simulink model "mech_stewart_js"  (Simulink 7.1)
settings: Solver=ode45  StartTime=0.0  StopTime=inf  RelTol=1e-3
PreLoadFcn:
  | mech_stewartplatform_dat
PostLoadFcn:
  | find_system(gcs,'FollowLinks', 'on', 'LookUnderMasks', 'all');
InitFcn:
  | find_system(gcs,'FollowLinks', 'on', 'LookUnderMasks', 'all');
values from neighbouring files (symbols this model uses):
  body_pts = pos_top' - height*[zeros(2,6);ones(1,6)]    [mech_stewart_studies_setup.m]    (also in mech_stewartplatform_dat.m)
  height = 2.0    (= 2)    [mech_stewart_studies_setup.m]    (also in mech_stewartplatform_dat.m)
  Kd = 4.5e4    (= 45000)    [mech_stewart_studies_setup.m]    (also in mech_stewartplatform_dat.m)
  Ki = 1e4    (= 10000)    [mech_stewart_studies_setup.m]    (also in mech_stewartplatform_dat.m)
  Kp = 2e6    (= 2000000)    [mech_stewart_studies_setup.m]    (also in mech_stewartplatform_dat.m)
  pos_base = []    [mech_stewart_studies_setup.m]    (also in mech_stewartplatform_dat.m)
  pos_top = [pos_top(6,:); pos_top(1:5,:)]    [mech_stewart_studies_setup.m]    (also in mech_stewartplatform_dat.m)
undefined symbols (not defined in the file or in its folder): lower_leg_mass, top_inertia, top_mass, upper_leg_mass
libraries: mblibv1 x9, simulink x6, mech_stewartplatform_leg x6, vrlib x1
Description:
  | Stewart Platform with Joystick Control
  | 
  | Stewart platform with external virtual reality joystick control.
settings Model: Creator=jwendlan  LastModifiedBy=batserve  ExtModeAutoUpdateStatusClock=off
settings DataIOCC: SignalLoggingName=sigsOut  OutputTimes=[0:0.01:50]
settings OptimizationCC: BooleanDataType=off  InlineInvariantSignals=on
settings DebuggingCC: SaveWithParameterizedLinksMsg=none  CheckExecutionContextPreStartOutputMsg=on  CheckExecutionContextRuntimeOutputMsg=on  SignalResolutionControl=TryResolveAllWithWarning  SolverPrmCheckMsg=none  MultiTaskDSMMsg=warning  MultiTaskCondExecSysMsg=none  SigSpecEnsureSampleTimeMsg=none  UnconnectedOutputMsg=none  StrictBusMsg=None
settings HardwareCC: TargetBitPerLong=64  TargetEndianess=LittleEndian  TargetWordSize=64  TargetHWDeviceType=MATLAB Host  ProdEqTarget=off
settings RTWCC: SystemTargetFile=rsim.tlc  TemplateMakefile=rsim_default_tmf  Description=Rapid Simulation Target  ProcessScript=rsim_make_rtw_hook  IncludeERTFirstTime=on
settings RSimTargetCC: TargetFcnLib=ansi_tfl_tmw.mat  TargetFunctionLibrary=ANSI_C  IsPILTarget=off  EnableShiftOperators=on  PortableWordSizes=off
settings SimMechanicsCC: VisOnUpdateDiagram=on  VisDuringSimulation=on

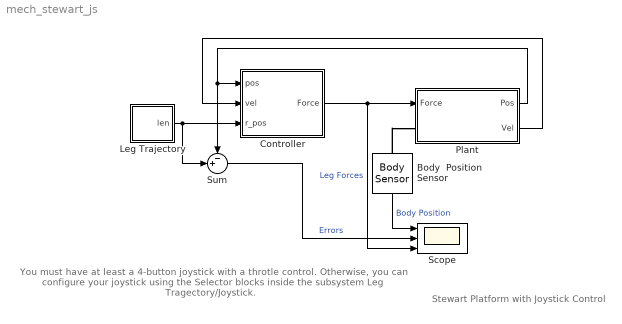
== system mech_stewart_js ==
  note: Stewart Platform
      | with Joystick Control
  note: You must have at least a 4-button
      | joystick with a throtle control.
      | Otherwise, you can configure
      | your joystick using the Selector
      | blocks inside the subsystem
      | Leg Tragectory/Joystick.
  Body  Position Sensor : mblibv1/Sensors &  Actuators/Body Sensor  Orientation=down  DialogController=MECH.DynMechDlgSource  SystemSampleTime=-1  PhysicalDomain=Mechanical  PortType=blob  Muxed=on  Pose=off  Angle=on  AngleUnits=deg  ArcVelocity=off  ArcVelocityUnits=deg/s  ArcAcceleration=off  ArcAccelerationUnits=deg/s^2  CoordPosition=on  CoordPositionUnits=m  Velocity=off  VelocityUnits=m/s  Acceleration=off  AccelerationUnits=m/s^2  Quaternion=on  QuaternionDT=off  QuaternionDDT=off  QuaternionUnits=off  OutputVector=[ 3 ]  ActiveIO=on  Width=3  DialogClass=MechanicalSensorBlock  ReferenceFrame=Absolute (World)
  Controller : Subsystem
  Leg Trajectory : Subsystem
  Plant : Subsystem
  Scope : Scope  NumInputPorts=3
      settings: Tag=OpenMeAtStartUp  YMin=-1~-1.1~-20000  YMax=3.5~1.1~40000
  Sum : Sum  Inputs=-+|  OutDataType=sfix(16)  OutScaling=2^0  SaturateOnIntegerOverflow=on  InputSameDT=on  OutDataTypeStr=Inherit: Same as first input
  wires:
  Controller/1(Force) -> Plant/1(Force), Scope/3  "Leg Forces"
  Body  Position Sensor/1 -> Scope/1  "Body Position"
  Sum/1 -> Scope/2  "Errors"
  Leg Trajectory/1(len) -> Controller/3(r_pos), Sum/2
  Plant/2(Vel) -> Controller/2(vel)
  Plant/1(Pos) -> Controller/1(pos), Sum/1
  connections:
  Body  Position Sensor/LConn1 -- Plant/LConn1

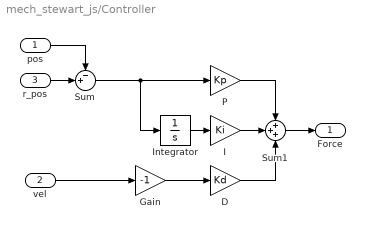
== system mech_stewart_js/Controller ==
  pos : Inport  OutDataType=sfix(16)  OutScaling=2^0
  vel : Inport  Port=2  OutDataType=sfix(16)  OutScaling=2^0
  r_pos : Inport  Port=3  OutDataType=sfix(16)  OutScaling=2^0
  D : Gain  Gain=Kd  ParameterDataType=sfix(16)  ParameterScaling=2^0  OutDataType=sfix(16)  OutScaling=2^0  SaturateOnIntegerOverflow=on  OutDataTypeStr=Inherit: Same as input  ParamDataTypeStr=Inherit: Same as input
  Gain : Gain  Gain=-1  ParameterDataType=sfix(16)  ParameterScaling=2^0  OutDataType=sfix(16)  OutScaling=2^0  SaturateOnIntegerOverflow=on  OutDataTypeStr=Inherit: Same as input  ParamDataTypeStr=Inherit: Same as input
  I : Gain  Gain=Ki  ParameterDataType=sfix(16)  ParameterScaling=2^0  OutDataType=sfix(16)  OutScaling=2^0  SaturateOnIntegerOverflow=on  OutDataTypeStr=Inherit: Same as input  ParamDataTypeStr=Inherit: Same as input
  Integrator : Integrator  InitialCondition=(upper_leg_mass+lower_leg_mass+(top_mass*1.3/6))*9.81/Ki  ZeroCross=off
  P : Gain  Gain=Kp  ParameterDataType=sfix(16)  ParameterScaling=2^0  OutDataType=sfix(16)  OutScaling=2^0  SaturateOnIntegerOverflow=on  OutDataTypeStr=Inherit: Same as input  ParamDataTypeStr=Inherit: Same as input
  Sum : Sum  Inputs=-+|  OutDataType=sfix(16)  OutScaling=2^0  SaturateOnIntegerOverflow=on  InputSameDT=on  OutDataTypeStr=Inherit: Same as first input
  Sum1 : Sum  Inputs=+++  OutDataType=sfix(16)  OutScaling=2^0  SaturateOnIntegerOverflow=on  InputSameDT=on  OutDataTypeStr=Inherit: Same as first input
  Force : Outport  OutDataType=sfix(16)  OutScaling=2^0
  wires:
  Sum/1 -> P/1, Integrator/1
  I/1 -> Sum1/2
  P/1 -> Sum1/1
  Integrator/1 -> I/1
  vel/1 -> Gain/1
  D/1 -> Sum1/3
  pos/1 -> Sum/1
  Sum1/1 -> Force/1
  r_pos/1 -> Sum/2
  Gain/1 -> D/1

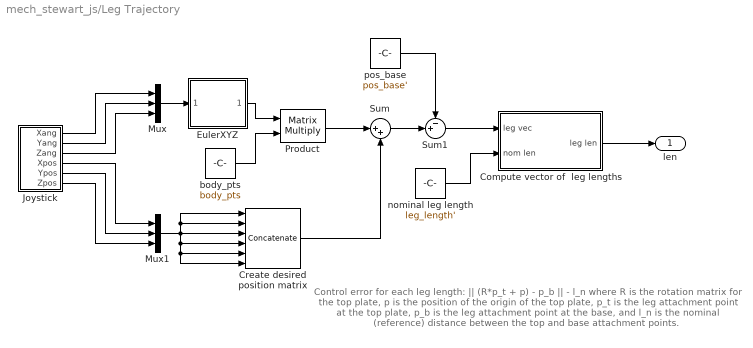
== system mech_stewart_js/Leg Trajectory ==
  note: Control error for each leg length:
      |
      |   || (R*p_t + p) - p_b || - l_n
      |
      | where R is the rotation matrix
      | for the top plate, p is the position
      | of the origin of the top plate, p_t
      | is the leg attachment point at the
      | top plate, p_b is the leg attachment
      | point at the base, and l_n is the
      | nominal (reference) distance between
      | the top and base attachment points.
  Compute vector of  leg lengths : Subsystem  TreatAsAtomicUnit=on
  Create desired position matrix : Concatenate  NumInputs=6  Mode=Multidimensional array  ConcatenateDimension=2
  EulerXYZ : Subsystem
      mask Type: EulerXYZ
      mask Description: Creates the EulerXYZ rotation matrix corresponding to body fixed rotations in the X, Y, and then Z. This matrix maps body vectors to world vectors.
      mask Help:
      | <p>This block determines the EulerXYZ matrix from a 3x1 euler angles in the X, Y, & Z directions. The matrix maps vectors the body axes to the inertial axes.</p>
      | 
      | <p>The block input and output contain more than one signal as described below.</p>
      | 
      | <p><H4>Block Vector Input - Euler XYZ angles</H4>
      |     <ul>
      |     <li>X angle</li>
      |     <li>Y angle</li>
      |     <li>Z angle</li>
      |    </ul>
      |    </p>
      | 
      | <p><H4>Block Matrix Output - XYZ Euler Matrix </H4>
      |     <ul>
      |    </ul>
      |    </p>
      mask Display: disp('Rotation\nMatrix')
  Joystick : Subsystem
  Mux : Mux  Inputs=3
  Mux1 : Mux  Inputs=3
  Product : Product  Multiplication=Matrix(*)  OutDataType=sfix(16)  OutScaling=2^0  SaturateOnIntegerOverflow=on  InputSameDT=on  OutDataTypeStr=Inherit: Same as first input
  Sum : Sum  Inputs=|++  OutDataType=sfix(16)  OutScaling=2^0  SaturateOnIntegerOverflow=on  InputSameDT=on  OutDataTypeStr=Inherit: Same as first input
  Sum1 : Sum  Inputs=-+|  OutDataType=sfix(16)  OutScaling=2^0  SaturateOnIntegerOverflow=on  InputSameDT=on  OutDataTypeStr=Inherit: Same as first input
  body_pts : Constant  Value=body_pts  VectorParams1D=off  OutDataType=sfix(16)  OutScaling=2^0
  nominal leg length : Constant  Value=leg_length'  VectorParams1D=off  OutDataType=sfix(16)  OutScaling=2^0
  pos_base : Constant  Value=pos_base'  VectorParams1D=off  OutDataType=sfix(16)  OutScaling=2^0
  len : Outport  OutDataType=sfix(16)  OutScaling=2^0
  wires:
  Joystick/6(Zpos) -> Mux1/3
  Joystick/5(Ypos) -> Mux1/2
  Joystick/4(Xpos) -> Mux1/1
  Joystick/2(Yang) -> Mux/2
  Joystick/1(Xang) -> Mux/1
  Joystick/3(Zang) -> Mux/3
  Compute vector of  leg lengths/1(leg len) -> len/1
  nominal leg length/1 -> Compute vector of  leg lengths/2(nom len)
  Sum1/1 -> Compute vector of  leg lengths/1(leg vec)
  Sum/1 -> Sum1/2
  pos_base/1 -> Sum1/1
  Create desired position matrix/1 -> Sum/2
  Mux1/1 -> Create desired position matrix/6, Create desired position matrix/5, Create desired position matrix/4, Create desired position matrix/2, Create desired position matrix/1, Create desired position matrix/3
  Product/1 -> Sum/1
  body_pts/1 -> Product/2
  EulerXYZ/1(EulerXYZ) -> Product/1
  Mux/1 -> EulerXYZ/1(x y z angles)

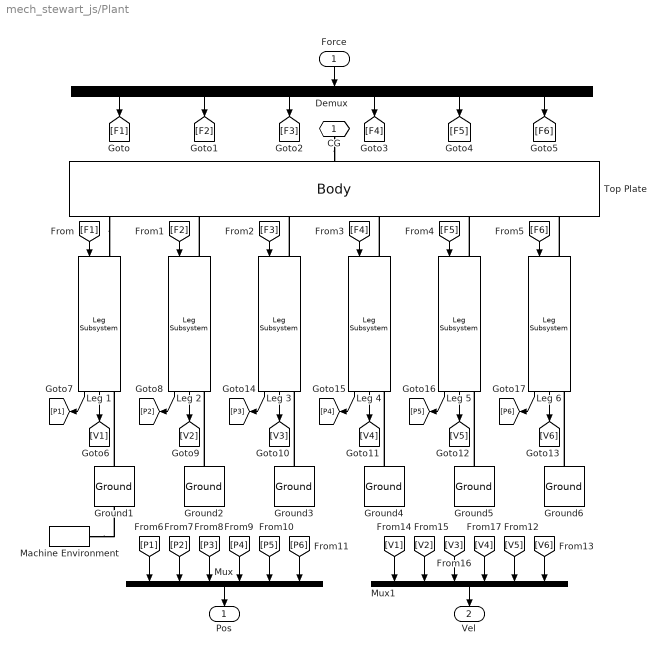
== system mech_stewart_js/Plant ==
  Force : Inport  Orientation=down  OutDataType=sfix(16)  OutScaling=2^0
  Demux : Demux  Orientation=down  Outputs=6
  Ground1 : mblibv1/Bodies/Ground  Orientation=up  DialogController=MECH.DynMechDlgSource  SystemSampleTime=-1  LeftPortType=env  RightPortType=workingframe  PhysicalDomain=Mechanical  DialogClass=GroundBlock  CoordPosition=pos_base(1,:)  CoordPositionUnits=m  StateVectorMgrId=-1  MachineId=[0 0]  ShowEnvPort=on
  Ground2 : mblibv1/Bodies/Ground  Orientation=up  DialogController=MECH.DynMechDlgSource  SystemSampleTime=-1  LeftPortType=env  RightPortType=workingframe  PhysicalDomain=Mechanical  DialogClass=GroundBlock  CoordPosition=pos_base(2,:)  CoordPositionUnits=m  StateVectorMgrId=-1  MachineId=[0 0]  ShowEnvPort=off
  Ground3 : mblibv1/Bodies/Ground  Orientation=up  DialogController=MECH.DynMechDlgSource  SystemSampleTime=-1  LeftPortType=env  RightPortType=workingframe  PhysicalDomain=Mechanical  DialogClass=GroundBlock  CoordPosition=pos_base(3,:)  CoordPositionUnits=m  StateVectorMgrId=-1  MachineId=[0 0]  ShowEnvPort=off
  Ground4 : mblibv1/Bodies/Ground  Orientation=up  DialogController=MECH.DynMechDlgSource  SystemSampleTime=-1  LeftPortType=env  RightPortType=workingframe  PhysicalDomain=Mechanical  DialogClass=GroundBlock  CoordPosition=pos_base(4,:)  CoordPositionUnits=m  StateVectorMgrId=-1  MachineId=[0 0]  ShowEnvPort=off
  Ground5 : mblibv1/Bodies/Ground  Orientation=up  DialogController=MECH.DynMechDlgSource  SystemSampleTime=-1  LeftPortType=env  RightPortType=workingframe  PhysicalDomain=Mechanical  DialogClass=GroundBlock  CoordPosition=pos_base(5,:)  CoordPositionUnits=m  StateVectorMgrId=-1  MachineId=[0 0]  ShowEnvPort=off
  Ground6 : mblibv1/Bodies/Ground  Orientation=up  DialogController=MECH.DynMechDlgSource  SystemSampleTime=-1  LeftPortType=env  RightPortType=workingframe  PhysicalDomain=Mechanical  DialogClass=GroundBlock  CoordPosition=pos_base(6,:)  CoordPositionUnits=m  StateVectorMgrId=-1  MachineId=[0 0]  ShowEnvPort=off
  Leg 1 : mech_stewartplatform_leg/Leg Subsystem  Orientation=down  SystemSampleTime=-1  ln=1
  Leg 2 : mech_stewartplatform_leg/Leg Subsystem  Orientation=down  SystemSampleTime=-1  ln=2
  Leg 3 : mech_stewartplatform_leg/Leg Subsystem  Orientation=down  SystemSampleTime=-1  ln=3
  Leg 4 : mech_stewartplatform_leg/Leg Subsystem  Orientation=down  SystemSampleTime=-1  ln=4
  Leg 5 : mech_stewartplatform_leg/Leg Subsystem  Orientation=down  SystemSampleTime=-1  ln=5
  Leg 6 : mech_stewartplatform_leg/Leg Subsystem  Orientation=down  SystemSampleTime=-1  ln=6
  Machine Environment : mblibv1/Bodies/Machine Environment  Tag=Factory ground  DialogController=MECH.DialogSource  SystemSampleTime=-1  PortType=env  PhysicalDomain=Mechanical  DialogTemplateClass=MECH.MachineEnvironment  SyncWhenCopied=off  Gravity=[0 0 -9.81]  GravityUnits=m/s^2  GravityAsSignal=off  Dimensionality=3D Only  AnalysisType=Forward dynamics  LinearAssemblyTolerance=1e-3  LinearAssemblyToleranceUnits=m  AngularAssemblyTolerance=1e-3  AngularAssemblyToleranceUnits=rad  ConstraintSolverType=Machine precision  ConstraintRelTolerance=1e-4  ConstraintAbsTolerance=1e-4  UseRobustSingularityHandling=on  RedundancyAnalysisToleranceType=Automatically select tolerance  RedundancyAnalysisTolerance=1e-14  StatePerturbationType=Adaptive  PerturbationSize=1e-3  VisualizeMachine=on
  Mux : Mux  Orientation=down  Inputs=6
  Mux1 : Mux  Orientation=down  Inputs=6
  Top Plate : mblibv1/Bodies/Body  Orientation=down  DialogController=MECH.DynMechDlgSource  PhysicalDomain=mechanical  SubClassName=Unknown  LeftPortType=workingframe  RightPortType=workingframe  LConnTagsString=CG  RConnTagsString=CS1|CS2|CS3|CS4|CS5|CS6  DialogClass=MechanicalBodyBlock  Mass=top_mass  MassUnits=kg  InertiaUnits=kg*m^2  Inertia=top_inertia  Shape=Cylinder  ShapeDims=[1 1]  ShapeUnits=m  ShapeUse=false  Density=1  DensityUnits=kg/m^3  DensityUse=false  GraphicsMode=1  BodyColor=[0.5 0.5 0.5]  GraphicsObj=[]  AttachedToCS=1  CG=Left$CG$[0 0 height]$WORLD$WORLD$m$[0 0 0]$Euler X-Y-Z$deg$WORLD$true  WorkingFrames=Right$CS1$pos_top(1,:)$WORLD$WORLD$m$[0 0 0]$Euler X-Y-Z$deg$WORLD$true#Right$CS2$pos_top(2,:)$WORLD$WORLD$m$[0 0 0]$Euler X-Y-Z$deg$WORLD$true#Right$CS3$pos_top(3,:)$WORLD$WORLD$m$[0 0 0]$Euler X-Y-Z$deg$WORLD$true#Right$CS4$pos_top(4,:)$WORLD$WORLD$m$[0 0 0]$Euler X-Y-Z$deg$WORLD$true#Right$CS5$pos_top(5,:)$WORLD$WORLD$m$[0 0 0]$Euler X-Y-Z$deg$WORLD$true#Right$CS6$pos_top(6,:)$WORLD$WORLD$m$[0 0 0]$Euler X-Y-Z$deg$WORLD$true  CGPos=[0 0 height]  CGRot=[0 0 0]  CS0Pos=[]  CS0Rot=[]  CS1Pos=pos_top(1,:)  CS1Rot=[0 0 0]  CS2Pos=pos_top(2,:)  CS2Rot=[0 0 0]  CS3Pos=pos_top(3,:)  CS3Rot=[0 0 0]  CS4Pos=pos_top(4,:)  CS4Rot=[0 0 0]  CS5Pos=pos_top(5,:)  CS5Rot=[0 0 0]  CS6Pos=pos_top(6,:)  CS6Rot=[0 0 0]  CS7Pos=[]  CS7Rot=[]  CS8Pos=[]  CS8Rot=[]  CS9Pos=[]  CS9Rot=[]  CS10Pos=[]  CS10Rot=[]  CS11Pos=[]  CS11Rot=[]  CS12Pos=[]  CS12Rot=[]  CS13Pos=[]  CS13Rot=[]  CS14Pos=[]  CS14Rot=[]  CS15Pos=[]  CS15Rot=[]  CS16Pos=[]  CS16Rot=[]  CS17Pos=[]  CS17Rot=[]  CS18Pos=[]  CS18Rot=[]  CS19Pos=[]  CS19Rot=[]  CS20Pos=[]  CS20Rot=[]
  CG : PMIOPort  Orientation=down  Port=1  Side=Left
  Pos : Outport  Orientation=down  OutDataType=sfix(16)  OutScaling=2^0
  Vel : Outport  Orientation=down  Port=2  OutDataType=sfix(16)  OutScaling=2^0
  wires:
  Force/1 -> Demux/1
  Mux/1 -> Pos/1
  Demux/1 -> [F1]
  Demux/2 -> [F2]
  Demux/3 -> [F3]
  Demux/4 -> [F4]
  Demux/5 -> [F5]
  Demux/6 -> [F6]
  [F1] -> Leg 1/1
  [F2] -> Leg 2/1
  [F3] -> Leg 3/1
  [F4] -> Leg 4/1
  [F5] -> Leg 5/1
  [F6] -> Leg 6/1
  Leg 1/2 -> [V1]
  Leg 1/1 -> [P1]
  Leg 2/2 -> [V2]
  Leg 3/2 -> [V3]
  Leg 4/2 -> [V4]
  Leg 5/2 -> [V5]
  Leg 6/2 -> [V6]
  Leg 2/1 -> [P2]
  Leg 3/1 -> [P3]
  Leg 4/1 -> [P4]
  Leg 5/1 -> [P5]
  Leg 6/1 -> [P6]
  [P1] -> Mux/1
  [P2] -> Mux/2
  [P3] -> Mux/3
  [P4] -> Mux/4
  [P5] -> Mux/5
  [P6] -> Mux/6
  [V1] -> Mux1/1
  [V2] -> Mux1/2
  [V3] -> Mux1/3
  [V4] -> Mux1/4
  [V5] -> Mux1/5
  [V6] -> Mux1/6
  Mux1/1 -> Vel/1
  connections:
  Top Plate/RConn1 -- Leg 1/LConn1
  Ground6/RConn1 -- Leg 6/RConn1
  Ground5/RConn1 -- Leg 5/RConn1
  Ground4/RConn1 -- Leg 4/RConn1
  Ground3/RConn1 -- Leg 3/RConn1
  Ground2/RConn1 -- Leg 2/RConn1
  Ground1/RConn1 -- Leg 1/RConn1
  Leg 2/LConn1 -- Top Plate/RConn2
  Leg 3/LConn1 -- Top Plate/RConn3
  Leg 4/LConn1 -- Top Plate/RConn4
  Leg 5/LConn1 -- Top Plate/RConn5
  Leg 6/LConn1 -- Top Plate/RConn6
  CG/RConn1 -- Top Plate/LConn1
  Machine Environment/RConn1 -- Ground1/LConn1

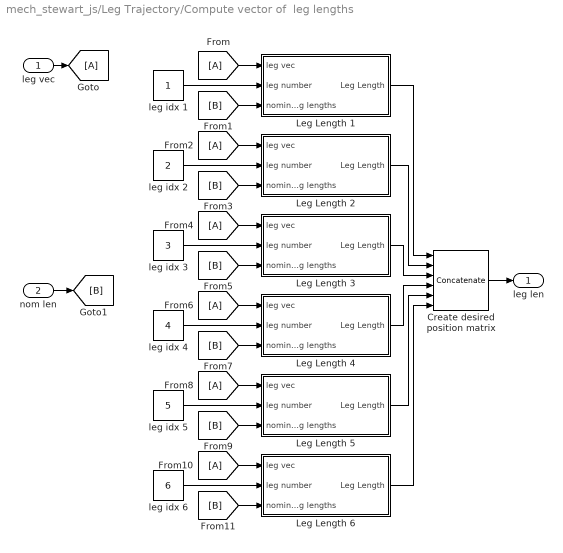
== system mech_stewart_js/Leg Trajectory/Compute vector of  leg lengths ==
  leg vec : Inport  OutDataType=sfix(16)  OutScaling=2^0
  nom len : Inport  Port=2  OutDataType=sfix(16)  OutScaling=2^0
  Create desired position matrix : Concatenate  NumInputs=6  Mode=Multidimensional array  ConcatenateDimension=2
  Leg Length 1 : Subsystem
  Leg Length 2 : Subsystem
  Leg Length 3 : Subsystem
  Leg Length 4 : Subsystem
  Leg Length 5 : Subsystem
  Leg Length 6 : Subsystem
  leg idx 1 : Constant  OutDataType=sfix(16)  OutScaling=2^0
  leg idx 2 : Constant  Value=2  OutDataType=sfix(16)  OutScaling=2^0
  leg idx 3 : Constant  Value=3  OutDataType=sfix(16)  OutScaling=2^0
  leg idx 4 : Constant  Value=4  OutDataType=sfix(16)  OutScaling=2^0
  leg idx 5 : Constant  Value=5  OutDataType=sfix(16)  OutScaling=2^0
  leg idx 6 : Constant  Value=6  OutDataType=sfix(16)  OutScaling=2^0
  leg len : Outport  OutDataType=sfix(16)  OutScaling=2^0
  wires:
  Leg Length 6/1(Leg Length) -> Create desired position matrix/6
  Leg Length 5/1(Leg Length) -> Create desired position matrix/5
  Leg Length 4/1(Leg Length) -> Create desired position matrix/4
  Leg Length 3/1(Leg Length) -> Create desired position matrix/3
  Leg Length 2/1(Leg Length) -> Create desired position matrix/2
  Leg Length 1/1(Leg Length) -> Create desired position matrix/1
  [B] -> Leg Length 6/3(nominal leg lengths)
  [A] -> Leg Length 6/1(leg vec)
  leg idx 6/1 -> Leg Length 6/2(leg number)
  [B] -> Leg Length 5/3(nominal leg lengths)
  [A] -> Leg Length 5/1(leg vec)
  leg idx 5/1 -> Leg Length 5/2(leg number)
  [B] -> Leg Length 4/3(nominal leg lengths)
  [A] -> Leg Length 4/1(leg vec)
  leg idx 4/1 -> Leg Length 4/2(leg number)
  [B] -> Leg Length 3/3(nominal leg lengths)
  [A] -> Leg Length 3/1(leg vec)
  leg idx 3/1 -> Leg Length 3/2(leg number)
  [B] -> Leg Length 2/3(nominal leg lengths)
  [A] -> Leg Length 2/1(leg vec)
  leg idx 2/1 -> Leg Length 2/2(leg number)
  [B] -> Leg Length 1/3(nominal leg lengths)
  nom len/1 -> [B]
  [A] -> Leg Length 1/1(leg vec)
  leg vec/1 -> [A]
  leg idx 1/1 -> Leg Length 1/2(leg number)
  Create desired position matrix/1 -> leg len/1

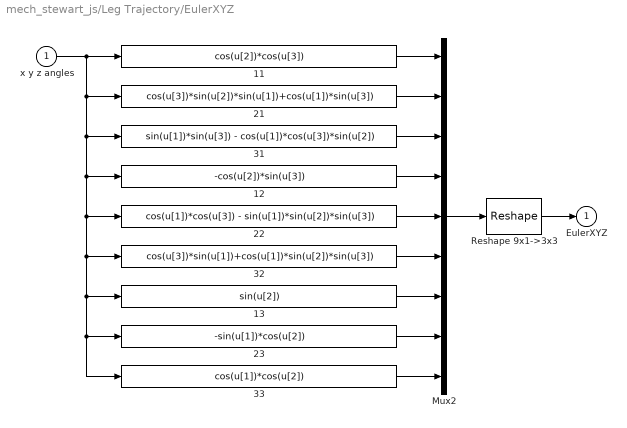
== system mech_stewart_js/Leg Trajectory/EulerXYZ ==
  x y z angles : Inport  OutDataType=sfix(16)  OutScaling=2^0
  11 : Fcn  Expr=cos(u[2])*cos(u[3])
  12 : Fcn  Expr=-cos(u[2])*sin(u[3])
  13 : Fcn  Expr=sin(u[2])
  21 : Fcn  Expr=cos(u[3])*sin(u[2])*sin(u[1])+cos(u[1])*sin(u[3])
  22 : Fcn  Expr=cos(u[1])*cos(u[3]) - sin(u[1])*sin(u[2])*sin(u[3])
  23 : Fcn  Expr=-sin(u[1])*cos(u[2])
  31 : Fcn  Expr=sin(u[1])*sin(u[3]) - cos(u[1])*cos(u[3])*sin(u[2])
  32 : Fcn  Expr=cos(u[3])*sin(u[1])+cos(u[1])*sin(u[2])*sin(u[3])
  33 : Fcn  Expr=cos(u[1])*cos(u[2])
  Mux2 : Mux  Inputs=9
  Reshape 9x1->3x3 : Reshape  OutputDimensionality=Customize  OutputDimensions=[3,3]
  EulerXYZ : Outport  OutDataType=sfix(16)  OutScaling=2^0  InitialOutput=0
  wires:
  Reshape 9x1->3x3/1 -> EulerXYZ/1
  Mux2/1 -> Reshape 9x1->3x3/1
  11/1 -> Mux2/1
  21/1 -> Mux2/2
  31/1 -> Mux2/3
  12/1 -> Mux2/4
  22/1 -> Mux2/5
  32/1 -> Mux2/6
  13/1 -> Mux2/7
  23/1 -> Mux2/8
  33/1 -> Mux2/9
  x y z angles/1 -> 11/1, 21/1, 31/1, 12/1, 22/1, 32/1, 13/1, 33/1, 23/1

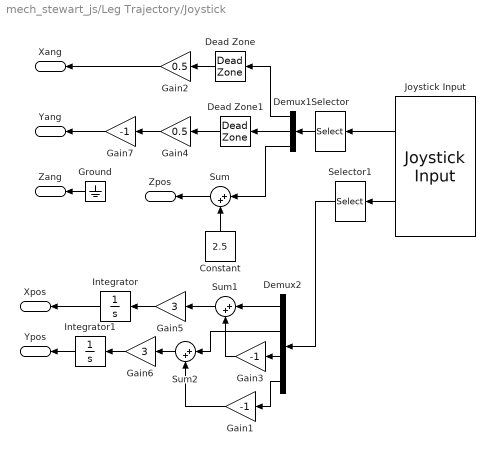
== system mech_stewart_js/Leg Trajectory/Joystick ==
  Constant : Constant  Orientation=up  Value=2.5  OutDataType=sfix(16)  OutScaling=2^0
  Dead Zone : DeadZone  Orientation=left  LowerValue=-0.05  UpperValue=0.05  ZeroCross=off  SaturateOnIntegerOverflow=on
  Dead Zone1 : DeadZone  Orientation=left  LowerValue=-0.05  UpperValue=0.05  ZeroCross=off  SaturateOnIntegerOverflow=on
  Demux1 : Demux  Orientation=left  Outputs=[1 1 1]
  Demux2 : Demux  Orientation=left
  Gain1 : Gain  Orientation=left  Gain=-1  ParameterDataType=sfix(16)  ParameterScaling=2^0  OutDataType=sfix(16)  OutScaling=2^0  SaturateOnIntegerOverflow=on  OutDataTypeStr=Inherit: Same as input  ParamDataTypeStr=Inherit: Same as input
  Gain2 : Gain  Orientation=left  Gain=0.5  ParameterDataType=sfix(16)  ParameterScaling=2^0  OutDataType=sfix(16)  OutScaling=2^0  SaturateOnIntegerOverflow=on  OutDataTypeStr=Inherit: Same as input  ParamDataTypeStr=Inherit: Same as input
  Gain3 : Gain  Orientation=left  Gain=-1  ParameterDataType=sfix(16)  ParameterScaling=2^0  OutDataType=sfix(16)  OutScaling=2^0  SaturateOnIntegerOverflow=on  OutDataTypeStr=Inherit: Same as input  ParamDataTypeStr=Inherit: Same as input
  Gain4 : Gain  Orientation=left  Gain=0.5  ParameterDataType=sfix(16)  ParameterScaling=2^0  OutDataType=sfix(16)  OutScaling=2^0  SaturateOnIntegerOverflow=on  OutDataTypeStr=Inherit: Same as input  ParamDataTypeStr=Inherit: Same as input
  Gain5 : Gain  Orientation=left  Gain=3  ParameterDataType=sfix(16)  ParameterScaling=2^0  OutDataType=sfix(16)  OutScaling=2^0  SaturateOnIntegerOverflow=on  OutDataTypeStr=Inherit: Same as input  ParamDataTypeStr=Inherit: Same as input
  Gain6 : Gain  Orientation=left  Gain=3  ParameterDataType=sfix(16)  ParameterScaling=2^0  OutDataType=sfix(16)  OutScaling=2^0  SaturateOnIntegerOverflow=on  OutDataTypeStr=Inherit: Same as input  ParamDataTypeStr=Inherit: Same as input
  Gain7 : Gain  Orientation=left  Gain=-1  ParameterDataType=sfix(16)  ParameterScaling=2^0  OutDataType=sfix(16)  OutScaling=2^0  SaturateOnIntegerOverflow=on  OutDataTypeStr=Inherit: Same as input  ParamDataTypeStr=Inherit: Same as input
  Ground : Ground  Orientation=left
  Integrator : Integrator  Orientation=left  ZeroCross=off
  Integrator1 : Integrator  Orientation=left  ZeroCross=off
  Joystick Input : vrlib/Joystick Input  Orientation=left  joyid=1  adjustports=on  forcefeed=off
  Selector : Selector  Orientation=left  IndexOptions=Index vector (dialog)  Indices=[1 2 3]  OutputSizes=1
  Selector1 : Selector  Orientation=left  IndexOptions=Index vector (dialog)  Indices=[1 2 4 3]  OutputSizes=1
  Sum : Sum  Orientation=left  Inputs=|++  OutDataType=sfix(16)  OutScaling=2^0  SaturateOnIntegerOverflow=on  InputSameDT=on  OutDataTypeStr=Inherit: Same as first input
  Sum1 : Sum  Orientation=left  Inputs=|++  OutDataType=sfix(16)  OutScaling=2^0  SaturateOnIntegerOverflow=on  InputSameDT=on  OutDataTypeStr=Inherit: Same as first input
  Sum2 : Sum  Orientation=left  Inputs=|++  OutDataType=sfix(16)  OutScaling=2^0  SaturateOnIntegerOverflow=on  InputSameDT=on  OutDataTypeStr=Inherit: Same as first input
  Xang : Outport  Orientation=left  OutDataType=sfix(16)  OutScaling=2^0
  Yang : Outport  Orientation=left  Port=2  OutDataType=sfix(16)  OutScaling=2^0
  Zang : Outport  Orientation=left  Port=3  OutDataType=sfix(16)  OutScaling=2^0
  Xpos : Outport  Orientation=left  Port=4  OutDataType=sfix(16)  OutScaling=2^0
  Ypos : Outport  Orientation=left  Port=5  OutDataType=sfix(16)  OutScaling=2^0
  Zpos : Outport  Orientation=left  Port=6  OutDataType=sfix(16)  OutScaling=2^0
  wires:
  Joystick Input/1 -> Selector/1
  Joystick Input/2 -> Selector1/1
  Demux1/3 -> Sum/1
  Constant/1 -> Sum/2
  Demux1/2 -> Dead Zone1/1
  Demux1/1 -> Dead Zone/1
  Gain3/1 -> Sum1/2
  Demux2/1 -> Sum1/1
  Sum1/1 -> Gain5/1
  Demux2/3 -> Gain3/1
  Gain1/1 -> Sum2/2
  Demux2/2 -> Sum2/1
  Sum2/1 -> Gain6/1
  Demux2/4 -> Gain1/1
  Sum/1 -> Zpos/1
  Integrator/1 -> Xpos/1
  Integrator1/1 -> Ypos/1
  Dead Zone/1 -> Gain2/1
  Dead Zone1/1 -> Gain4/1
  Ground/1 -> Zang/1
  Gain2/1 -> Xang/1
  Gain4/1 -> Gain7/1
  Gain5/1 -> Integrator/1
  Gain6/1 -> Integrator1/1
  Gain7/1 -> Yang/1
  Selector/1 -> Demux1/1
  Selector1/1 -> Demux2/1

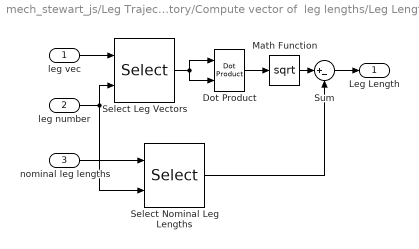
== system mech_stewart_js/Leg Trajectory/Compute vector of  leg lengths/Leg Length 1 ==
  leg vec : Inport  OutDataType=sfix(16)  OutScaling=2^0
  leg number : Inport  Port=2  OutDataType=sfix(16)  OutScaling=2^0
  nominal leg lengths : Inport  Port=3  OutDataType=sfix(16)  OutScaling=2^0
  Dot Product : simulink/Math Operations/Dot Product  OutDataType=sfix(16)  OutScaling=2^-10  DoSatur=off
  Math Function : Math  Operator=sqrt  OutDataType=sfix(16)  OutScaling=2^0  SaturateOnIntegerOverflow=on
  Select Leg Vectors : Selector  NumberOfDimensions=2  InputPortWidth=3  IndexOptions=Select all,Index vector (port)  Indices=-1,1  OutputSizes=1
  Select Nominal Leg Lengths : Selector  InputPortWidth=6  IndexOptions=Index vector (port)  Indices=[1 3]  OutputSizes=1
  Sum : Sum  Inputs=|+-  OutDataType=sfix(16)  OutScaling=2^0  SaturateOnIntegerOverflow=on  InputSameDT=on  OutDataTypeStr=Inherit: Same as first input
  Leg Length : Outport  OutDataType=sfix(16)  OutScaling=2^0
  wires:
  nominal leg lengths/1 -> Select Nominal Leg Lengths/1
  Sum/1 -> Leg Length/1
  leg vec/1 -> Select Leg Vectors/1
  leg number/1 -> Select Leg Vectors/2, Select Nominal Leg Lengths/2
  Dot Product/1 -> Math Function/1
  Select Leg Vectors/1 -> Dot Product/1, Dot Product/2
  Math Function/1 -> Sum/1
  Select Nominal Leg Lengths/1 -> Sum/2

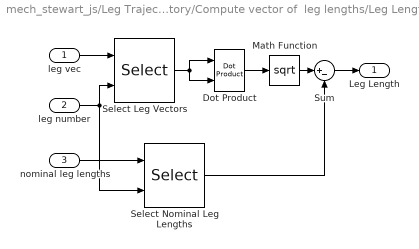
== system mech_stewart_js/Leg Trajectory/Compute vector of  leg lengths/Leg Length 2 ==
  leg vec : Inport  OutDataType=sfix(16)  OutScaling=2^0
  leg number : Inport  Port=2  OutDataType=sfix(16)  OutScaling=2^0
  nominal leg lengths : Inport  Port=3  OutDataType=sfix(16)  OutScaling=2^0
  Dot Product : simulink/Math Operations/Dot Product  OutDataType=sfix(16)  OutScaling=2^-10  DoSatur=off
  Math Function : Math  Operator=sqrt  OutDataType=sfix(16)  OutScaling=2^0  SaturateOnIntegerOverflow=on
  Select Leg Vectors : Selector  NumberOfDimensions=2  InputPortWidth=3  IndexOptions=Select all,Index vector (port)  Indices=-1,1  OutputSizes=1
  Select Nominal Leg Lengths : Selector  InputPortWidth=6  IndexOptions=Index vector (port)  Indices=[1 3]  OutputSizes=1
  Sum : Sum  Inputs=|+-  OutDataType=sfix(16)  OutScaling=2^0  SaturateOnIntegerOverflow=on  InputSameDT=on  OutDataTypeStr=Inherit: Same as first input
  Leg Length : Outport  OutDataType=sfix(16)  OutScaling=2^0
  wires:
  nominal leg lengths/1 -> Select Nominal Leg Lengths/1
  Sum/1 -> Leg Length/1
  leg vec/1 -> Select Leg Vectors/1
  leg number/1 -> Select Leg Vectors/2, Select Nominal Leg Lengths/2
  Dot Product/1 -> Math Function/1
  Select Leg Vectors/1 -> Dot Product/1, Dot Product/2
  Math Function/1 -> Sum/1
  Select Nominal Leg Lengths/1 -> Sum/2

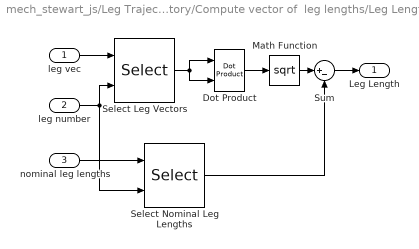
== system mech_stewart_js/Leg Trajectory/Compute vector of  leg lengths/Leg Length 3 ==
  leg vec : Inport  OutDataType=sfix(16)  OutScaling=2^0
  leg number : Inport  Port=2  OutDataType=sfix(16)  OutScaling=2^0
  nominal leg lengths : Inport  Port=3  OutDataType=sfix(16)  OutScaling=2^0
  Dot Product : simulink/Math Operations/Dot Product  OutDataType=sfix(16)  OutScaling=2^-10  DoSatur=off
  Math Function : Math  Operator=sqrt  OutDataType=sfix(16)  OutScaling=2^0  SaturateOnIntegerOverflow=on
  Select Leg Vectors : Selector  NumberOfDimensions=2  InputPortWidth=3  IndexOptions=Select all,Index vector (port)  Indices=-1,1  OutputSizes=1
  Select Nominal Leg Lengths : Selector  InputPortWidth=6  IndexOptions=Index vector (port)  Indices=[1 3]  OutputSizes=1
  Sum : Sum  Inputs=|+-  OutDataType=sfix(16)  OutScaling=2^0  SaturateOnIntegerOverflow=on  InputSameDT=on  OutDataTypeStr=Inherit: Same as first input
  Leg Length : Outport  OutDataType=sfix(16)  OutScaling=2^0
  wires:
  nominal leg lengths/1 -> Select Nominal Leg Lengths/1
  Sum/1 -> Leg Length/1
  leg vec/1 -> Select Leg Vectors/1
  leg number/1 -> Select Leg Vectors/2, Select Nominal Leg Lengths/2
  Dot Product/1 -> Math Function/1
  Select Leg Vectors/1 -> Dot Product/1, Dot Product/2
  Math Function/1 -> Sum/1
  Select Nominal Leg Lengths/1 -> Sum/2

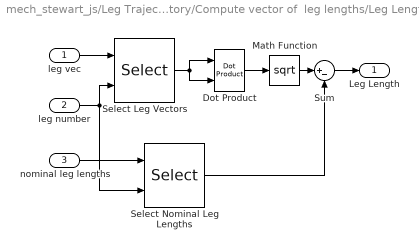
== system mech_stewart_js/Leg Trajectory/Compute vector of  leg lengths/Leg Length 4 ==
  leg vec : Inport  OutDataType=sfix(16)  OutScaling=2^0
  leg number : Inport  Port=2  OutDataType=sfix(16)  OutScaling=2^0
  nominal leg lengths : Inport  Port=3  OutDataType=sfix(16)  OutScaling=2^0
  Dot Product : simulink/Math Operations/Dot Product  OutDataType=sfix(16)  OutScaling=2^-10  DoSatur=off
  Math Function : Math  Operator=sqrt  OutDataType=sfix(16)  OutScaling=2^0  SaturateOnIntegerOverflow=on
  Select Leg Vectors : Selector  NumberOfDimensions=2  InputPortWidth=3  IndexOptions=Select all,Index vector (port)  Indices=-1,1  OutputSizes=1
  Select Nominal Leg Lengths : Selector  InputPortWidth=6  IndexOptions=Index vector (port)  Indices=[1 3]  OutputSizes=1
  Sum : Sum  Inputs=|+-  OutDataType=sfix(16)  OutScaling=2^0  SaturateOnIntegerOverflow=on  InputSameDT=on  OutDataTypeStr=Inherit: Same as first input
  Leg Length : Outport  OutDataType=sfix(16)  OutScaling=2^0
  wires:
  nominal leg lengths/1 -> Select Nominal Leg Lengths/1
  Sum/1 -> Leg Length/1
  leg vec/1 -> Select Leg Vectors/1
  leg number/1 -> Select Leg Vectors/2, Select Nominal Leg Lengths/2
  Dot Product/1 -> Math Function/1
  Select Leg Vectors/1 -> Dot Product/1, Dot Product/2
  Math Function/1 -> Sum/1
  Select Nominal Leg Lengths/1 -> Sum/2

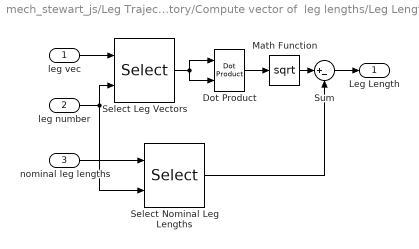
== system mech_stewart_js/Leg Trajectory/Compute vector of  leg lengths/Leg Length 5 ==
  leg vec : Inport  OutDataType=sfix(16)  OutScaling=2^0
  leg number : Inport  Port=2  OutDataType=sfix(16)  OutScaling=2^0
  nominal leg lengths : Inport  Port=3  OutDataType=sfix(16)  OutScaling=2^0
  Dot Product : simulink/Math Operations/Dot Product  OutDataType=sfix(16)  OutScaling=2^-10  DoSatur=off
  Math Function : Math  Operator=sqrt  OutDataType=sfix(16)  OutScaling=2^0  SaturateOnIntegerOverflow=on
  Select Leg Vectors : Selector  NumberOfDimensions=2  InputPortWidth=3  IndexOptions=Select all,Index vector (port)  Indices=-1,1  OutputSizes=1
  Select Nominal Leg Lengths : Selector  InputPortWidth=6  IndexOptions=Index vector (port)  Indices=[1 3]  OutputSizes=1
  Sum : Sum  Inputs=|+-  OutDataType=sfix(16)  OutScaling=2^0  SaturateOnIntegerOverflow=on  InputSameDT=on  OutDataTypeStr=Inherit: Same as first input
  Leg Length : Outport  OutDataType=sfix(16)  OutScaling=2^0
  wires:
  nominal leg lengths/1 -> Select Nominal Leg Lengths/1
  Sum/1 -> Leg Length/1
  leg vec/1 -> Select Leg Vectors/1
  leg number/1 -> Select Leg Vectors/2, Select Nominal Leg Lengths/2
  Dot Product/1 -> Math Function/1
  Select Leg Vectors/1 -> Dot Product/1, Dot Product/2
  Math Function/1 -> Sum/1
  Select Nominal Leg Lengths/1 -> Sum/2

== system mech_stewart_js/Leg Trajectory/Compute vector of  leg lengths/Leg Length 6 ==
  leg vec : Inport  OutDataType=sfix(16)  OutScaling=2^0
  leg number : Inport  Port=2  OutDataType=sfix(16)  OutScaling=2^0
  nominal leg lengths : Inport  Port=3  OutDataType=sfix(16)  OutScaling=2^0
  Dot Product : simulink/Math Operations/Dot Product  OutDataType=sfix(16)  OutScaling=2^-10  DoSatur=off
  Math Function : Math  Operator=sqrt  OutDataType=sfix(16)  OutScaling=2^0  SaturateOnIntegerOverflow=on
  Select Leg Vectors : Selector  NumberOfDimensions=2  InputPortWidth=3  IndexOptions=Select all,Index vector (port)  Indices=-1,1  OutputSizes=1
  Select Nominal Leg Lengths : Selector  InputPortWidth=6  IndexOptions=Index vector (port)  Indices=[1 3]  OutputSizes=1
  Sum : Sum  Inputs=|+-  OutDataType=sfix(16)  OutScaling=2^0  SaturateOnIntegerOverflow=on  InputSameDT=on  OutDataTypeStr=Inherit: Same as first input
  Leg Length : Outport  OutDataType=sfix(16)  OutScaling=2^0
  wires:
  nominal leg lengths/1 -> Select Nominal Leg Lengths/1
  Sum/1 -> Leg Length/1
  leg vec/1 -> Select Leg Vectors/1
  leg number/1 -> Select Leg Vectors/2, Select Nominal Leg Lengths/2
  Dot Product/1 -> Math Function/1
  Select Leg Vectors/1 -> Dot Product/1, Dot Product/2
  Math Function/1 -> Sum/1
  Select Nominal Leg Lengths/1 -> Sum/2
